simulink model "worldGenerator"  (R2016b)
settings: Solver=FixedStepAuto  StartTime=0.0  StopTime=inf  RelTol=1e-3
model workspace (MAT data in the model file):
  SL_ROS_VariableLengthArrays_MaxSizes : struct (value not decoded)
libraries: robotlib x2
(part 2 of 2)

== matlab function worldGenerator/store_array ==
  data: x_a input size=20; y_a input size=20; counter input; counter_next output; x_aNext output size=20; y_aNext output size=20; class_next output size=20; class input size=20; Points input
function [counter_next, x_aNext,y_aNext, class_next] = fcn(x_a, y_a, counter, class, Points)
size = 0;
tmpX = 0;
tmpY = 0;
for k = 1:length(Points(:))
    if(double(Points(k).X) == tmpX && double(Points(k).Y) == tmpY)
        break;
    else
        size = size + 1;
        tmpX = double(Points(k).X);
        tmpY = double(Points(k).Y);
    end
end
x_pose = 0;
y_pose = 0;

x_test = zeros(32, 1);
y_test = zeros(32, 1);

if(size ~= 0)
    x_max = double(Points(1).X);
    x_min = double(Points(1).X);
    y_max = double(Points(1).Y);
    y_min = double(Points(1).Y);
else
     x_max = 0;
    x_min = 0;
    y_max = 0;
    y_min = 0;
end
sameNumX = 0;
sameNumY = 0;
for i = 1:size
    x_test(i) = double(Points(i).X);
    y_test(i) = double(Points(i).Y);
    x_pose = x_pose + double(Points(i).X);
    y_pose = y_pose + double(Points(i).Y);
    if(ismember(double(Points(i).X), x_test(:)))
        sameNumX = sameNumX + 1;
    end
    if(ismember(double(Points(i).Y), y_test(:)))
        sameNumY = sameNumY + 1;
    end
    if(i ~= 1)
        if(double(Points(i).X) > x_max)
            x_max = double(Points(i).X);
        end
        if(double(Points(i).X) < x_min)
            x_min = double(Points(i).X);
        end
        if(double(Points(i).Y) > y_max)
            y_max = double(Points(i).Y);
        end
        if(double(Points(i).Y) < y_min)
            y_min = double(Points(i).Y);
        end        
    end
    
    
end

if(size == 0)
    x_pose = 0;
    y_pose = 0;
else
    x_pose = x_pose / size;
    y_pose = y_pose / size;
end


if(counter == 0 && (x_pose ~= 0 || y_pose ~= 0))
    class_next = class;
    x_aNext = x_a;
    y_aNext = y_a;
    x_a(counter+1) = x_pose;
    y_a(counter+1) = y_pose;
    % Construction Barrier
    if(abs(x_max - x_min) < 0.5 && abs(y_max - y_min) < 0.5)
        class(counter + 1) = 1;
    % Box
    elseif((sameNumX  >= 2 || sameNumY >= 2) && size < 16)
        class(counter + 1) = 2;
    % Sphere
    elseif((sameNumX ~= 0 && sameNumY ~= 0) && abs(x_max - x_min) >= 0.5 && abs(y_max - y_min) >= 0.5)
        class(counter + 1) = 3;
    % Jersey Barrier
    elseif(size >= 16)
        class(counter + 1) = 4;
    else
        class(counter + 1) = 2;
    end 
    x_aNext = x_a;
    y_aNext = y_a;
    class_next = class;
    counter = counter + 1;
elseif(x_pose ~= 0 || y_pose ~= 0)
    flag = false;
    for i = 1:counter
        if(abs(x_a(i)-x_pose) <= 3 && abs(y_a(i)-y_pose) <= 3)
            flag = true;
            break;
        end
    end
    if(flag && size >= 16)
        class(counter) = 4;
    end
    if(flag == false)
        % Construction Barrier
        if(sameNumX ~= 0 && sameNumY ~= 0 && abs(x_max - x_min) < 0.5 && abs(y_max - y_min) < 0.5)
            class(counter + 1) = 3;
        % Box
        elseif((sameNumX  >= 2 || sameNumY >= 2) && size < 16)
            class(counter + 1) = 1;
        % Sphere
        elseif((sameNumX ~= 0 && sameNumY ~= 0) && abs(x_max - x_min) >= 0.5 && abs(y_max - y_min) >= 0.5)
            class(counter + 1) = 2;
        % Jersey Barrier
        elseif(size >= 16)
            class(counter + 1) = 4;
        else
            class(counter + 1) = 3;
        end
        x_a(counter+1) = x_pose;
        y_a(counter+1) = y_pose;
        counter = counter + 1;
    end
    class_next = class;
    x_aNext = x_a;
    y_aNext = y_a;
else
    class_next = class;
    x_aNext = x_a;
    y_aNext = y_a;
end
counter_next = counter;
